simulink model "model245"  (R2024b)
settings: Solver=VariableStepAuto  StartTime=0.0  StopTime=10.0  RelTol=1e-3
settings Model: Creator=Xist  LastModifiedBy=Xist

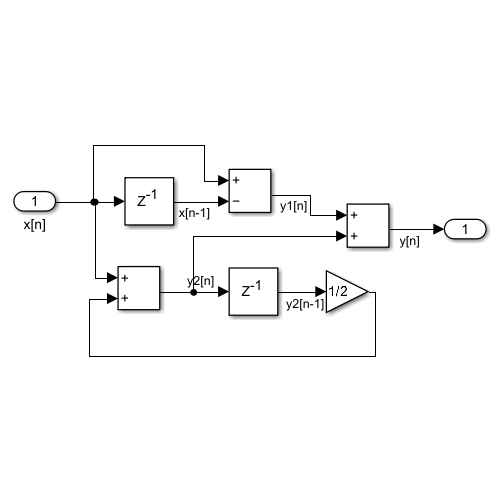
[thumbnail: Simulink's stored preview of the top-level diagram]
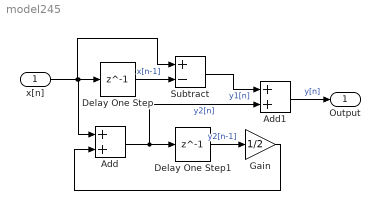
== system model245 ==
  x[n] : Inport
  Add : Sum
  Add1 : Sum
  Delay One Step : Delay  DelayLength=1
  Delay One Step1 : Delay  DelayLength=1
  Gain : Gain  Gain=1/2
  Subtract : Sum  Inputs=+-
  Output : Outport
  wires:
  x[n]/1 -> Add/1, Delay One Step/1, Subtract/1
  Subtract/1 -> Add1/1  "y1[n]"
  Delay One Step/1 -> Subtract/2  "x[n-1]"
  Delay One Step1/1 -> Gain/1  "y2[n-1]"
  Add/1 -> Add1/2, Delay One Step1/1  "y2[n]"
  Gain/1 -> Add/2
  Add1/1 -> Output/1  "y[n]"
